simulink model "pi_control_with_parameter_change"  (R2023b)
settings: Solver=VariableStepAuto  StartTime=0.0  StopTime=10.0  RelTol=1e-3
settings Model: Creator=kijun  LastModifiedBy=kijun

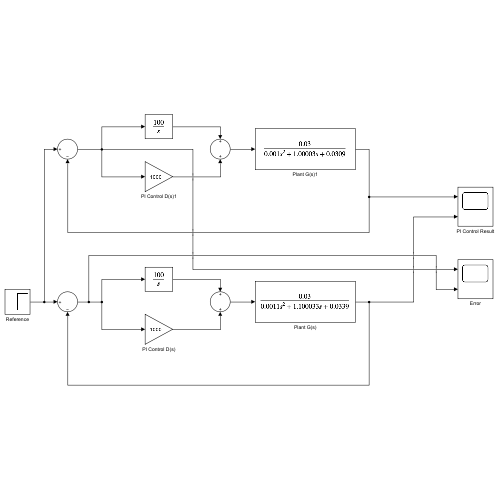
[thumbnail: Simulink's stored preview of the top-level diagram]
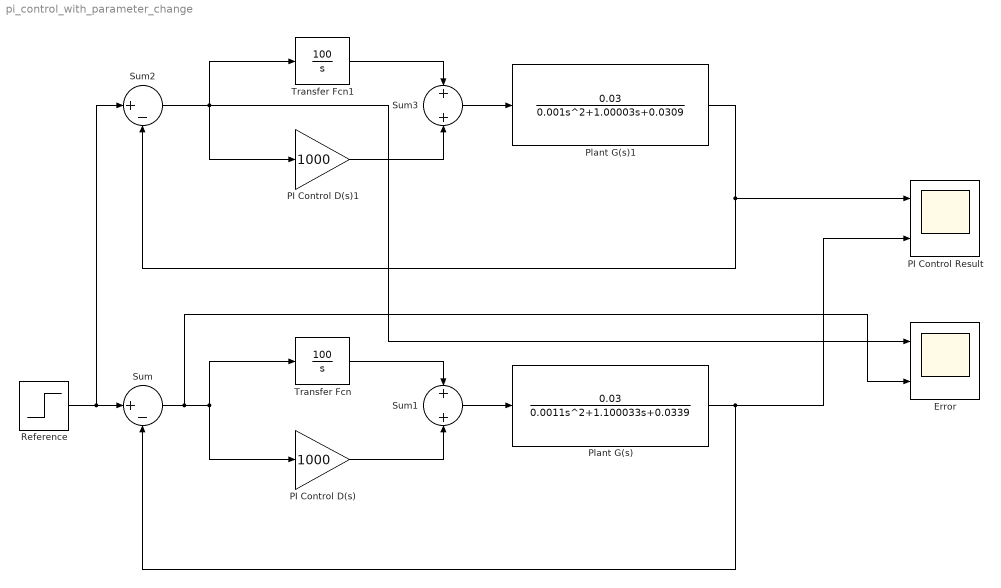
== system pi_control_with_parameter_change ==
  Error : Scope  NumInputPorts=2
  PI Control D(s) : Gain  Gain=1000
  PI Control D(s)1 : Gain  Gain=1000
  PI Control Result : Scope  NumInputPorts=2
  Plant G(s) : TransferFcn  Numerator=[0.03]  Denominator=[0.0011 1.100033 0.0339]
  Plant G(s)1 : TransferFcn  Numerator=[0.03]  Denominator=[0.001 1.00003 0.0309]
  Reference : Step  Time=0  SampleTime=0
  Sum : Sum  Inputs=|+-
  Sum1 : Sum  Inputs=+|+
  Sum2 : Sum  Inputs=|+-
  Sum3 : Sum  Inputs=+|+
  Transfer Fcn : TransferFcn  Numerator=100  Denominator=[1 0]
  Transfer Fcn1 : TransferFcn  Numerator=100  Denominator=[1 0]
  wires:
  Sum1/1 -> Plant G(s)/1
  PI Control D(s)/1 -> Sum1/2
  Plant G(s)/1 -> PI Control Result/2, Sum/2
  Sum/1 -> Error/2, PI Control D(s)/1, Transfer Fcn/1
  Transfer Fcn/1 -> Sum1/1
  Sum3/1 -> Plant G(s)1/1
  PI Control D(s)1/1 -> Sum3/2
  Transfer Fcn1/1 -> Sum3/1
  Sum2/1 -> Error/1, PI Control D(s)1/1, Transfer Fcn1/1
  Reference/1 -> Sum2/1, Sum/1
  Plant G(s)1/1 -> PI Control Result/1, Sum2/2
